simulink model "dlbsDocs"  (R2025b)
settings: Solver=VariableStepAuto  StartTime=0.0  StopTime=10.0  RelTol=1e-3
libraries: dlbsBlockExtractGradientGF x2, dlbsBlockInsertGradientGF x2, dlbsBlockBias x1, dlbsBlockSquare x1, dlbsBlockSpecifyDimensions x1
settings Model: Creator=lt6037  LastModifiedBy=lt6037

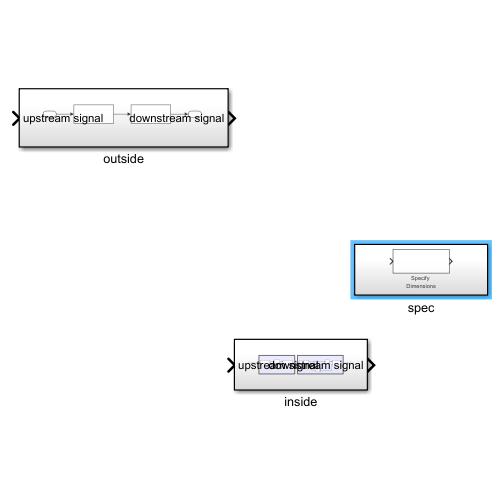
[thumbnail: Simulink's stored preview of the top-level diagram]
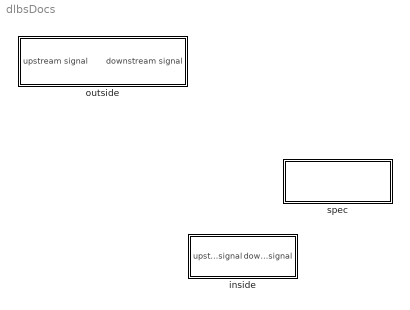
== system dlbsDocs ==
  inside : Subsystem
  outside : Subsystem
  spec : Subsystem

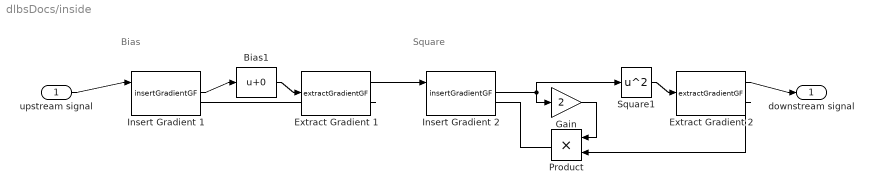
== system dlbsDocs/inside ==
  note: Square
  note: Bias
  upstream signal : Inport
  Bias1 : Bias  SaturateOnIntegerOverflow=off
  Extract Gradient 2 : dlbsBlockExtractGradientGF/extractGradientGF
  Extract Gradient 1 : dlbsBlockExtractGradientGF/extractGradientGF
  Gain : Gain  Gain=2
  Insert Gradient 1 : dlbsBlockInsertGradientGF/insertGradientGF
  Insert Gradient 2 : dlbsBlockInsertGradientGF/insertGradientGF
  Product : Product
  Square1 : Math  Operator=square
  downstream signal : Outport
  wires:
  Extract Gradient 2/1 -> downstream signal/1
  Extract Gradient 1/2 -> Insert Gradient 1/2
  Insert Gradient 1/1 -> Bias1/1
  Bias1/1 -> Extract Gradient 1/1
  upstream signal/1 -> Insert Gradient 1/1
  Gain/1 -> Product/1
  Insert Gradient 2/1 -> Square1/1, Gain/1
  Square1/1 -> Extract Gradient 2/1
  Extract Gradient 2/2 -> Product/2
  Product/1 -> Insert Gradient 2/2
  Extract Gradient 1/1 -> Insert Gradient 2/1

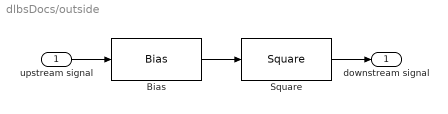
== system dlbsDocs/outside ==
  upstream signal : Inport
  Bias : dlbsBlockBias/Bias  Bias=0
  Square : dlbsBlockSquare/Square
  downstream signal : Outport
  wires:
  upstream signal/1 -> Bias/1
  Bias/1 -> Square/1
  Square/1 -> downstream signal/1

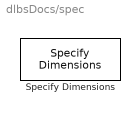
== system dlbsDocs/spec ==
  Specify Dimensions : dlbsBlockSpecifyDimensions/Specify Dimensions  value_size=[3,1,4]  grad_size=[3,1,4]
